simulink model "KERS_System_versione2"  (R2020a)
settings: Solver=VariableStepAuto  StartTime=0.0  StopTime=20  RelTol=1e-3
values from neighbouring files (symbols this model uses):
  Beta1 = 0.02    [Parameters.m]
  Beta2 = 0    [Parameters.m]
  Cx = 0.9    [Parameters.m]
  h = 0.1    [Parameters.m]
  Je = 0.3    [Kers_Energy_Characteristics.m]    (also in Kers_Energy_Characteristics_BiVariate.m; Parameters.m)
  Jf = 0.026    [Kers_Energy_Characteristics.m]    (also in Kers_Energy_Characteristics_BiVariate.m; Parameters.m)
  Jw = 1/2*(Rw^2*Mw)    (= 0.49005)    [Kers_Energy_Characteristics.m]    (also in Kers_Energy_Characteristics_BiVariate.m; Parameters.m)
  k = 0.01    [Parameters.m]
  M = 700    [Kers_Energy_Characteristics.m]    (also in Kers_Energy_Characteristics_BiVariate.m; Parameters.m)
  r_i = 0.05    [Parameters.m]
  r_o = 0.1    [Parameters.m]
  rho = Jeq^2*Jc/((Jc+Jeq)^2*gamma(i))    [Kers_Energy_Characteristics.m]    (also in Parameters.m = 1.2)
  rho_fw = 2267    [Parameters.m]
  Rw = 0.33    [Kers_Energy_Characteristics.m]    (also in Kers_Energy_Characteristics_BiVariate.m; Parameters.m)
  Sf = 1.5    [Parameters.m]
  tau1 = 1/3.08    (= 0.324675324675)    [Kers_Energy_Characteristics.m]    (also in Kers_Energy_Characteristics_BiVariate.m; Parameters.m)
  tau2 = 1/2.18    (= 0.45871559633)    [Kers_Energy_Characteristics.m]    (also in Kers_Energy_Characteristics_BiVariate.m; Parameters.m)
  tau3 = 1/1.63    (= 0.613496932515)    [Kers_Energy_Characteristics.m]    (also in Kers_Energy_Characteristics_BiVariate.m; Parameters.m)
  tau4 = 1/1.29    (= 0.77519379845)    [Kers_Energy_Characteristics.m]    (also in Kers_Energy_Characteristics_BiVariate.m; Parameters.m)
  tau5 = 1/1.03    (= 0.970873786408)    [Kers_Energy_Characteristics.m]    (also in Kers_Energy_Characteristics_BiVariate.m; Parameters.m)
  tau6 = 1/0.84    (= 1.19047619048)    [Kers_Energy_Characteristics.m]    (also in Kers_Energy_Characteristics_BiVariate.m; Parameters.m)
  tau7 = 1/0.69    (= 1.44927536232)    [Kers_Energy_Characteristics.m]    (also in Kers_Energy_Characteristics_BiVariate.m; Parameters.m)
  tauf = 1/4.38    (= 0.228310502283)    [Kers_Energy_Characteristics.m]    (also in Kers_Energy_Characteristics_BiVariate.m; Parameters.m)
  V1max = tauf*tau1*Rw*Wmax    (= 23.0528375734)    [Kers_Energy_Characteristics.m]    (also in Kers_Energy_Characteristics_BiVariate.m; Parameters.m)
  V2max = tauf*tau2*Rw*Wmax    (= 32.5700640945)    [Kers_Energy_Characteristics.m]    (also in Kers_Energy_Characteristics_BiVariate.m; Parameters.m)
  V3max = tauf*tau3*Rw*Wmax    (= 43.5599630221)    [Kers_Energy_Characteristics.m]    (also in Kers_Energy_Characteristics_BiVariate.m; Parameters.m)
  V4max = tauf*tau4*Rw*Wmax    (= 55.0408835085)    [Kers_Energy_Characteristics.m]    (also in Kers_Energy_Characteristics_BiVariate.m; Parameters.m)
  V5max = tauf*tau5*Rw*Wmax    (= 68.9346987631)    [Kers_Energy_Characteristics.m]    (also in Kers_Energy_Characteristics_BiVariate.m; Parameters.m)
  V6max = tauf*tau6*Rw*Wmax    (= 84.5270711024)    [Kers_Energy_Characteristics.m]    (also in Kers_Energy_Characteristics_BiVariate.m; Parameters.m)
  w_fw_max = 6283    [Parameters.m]
libraries: simulink x1
settings Model: Creator=Federico Kieffer  LastModifiedBy=Luca
settings SFSimCC: CustomCodeUndefinedFunction=UseInterfaceOnly

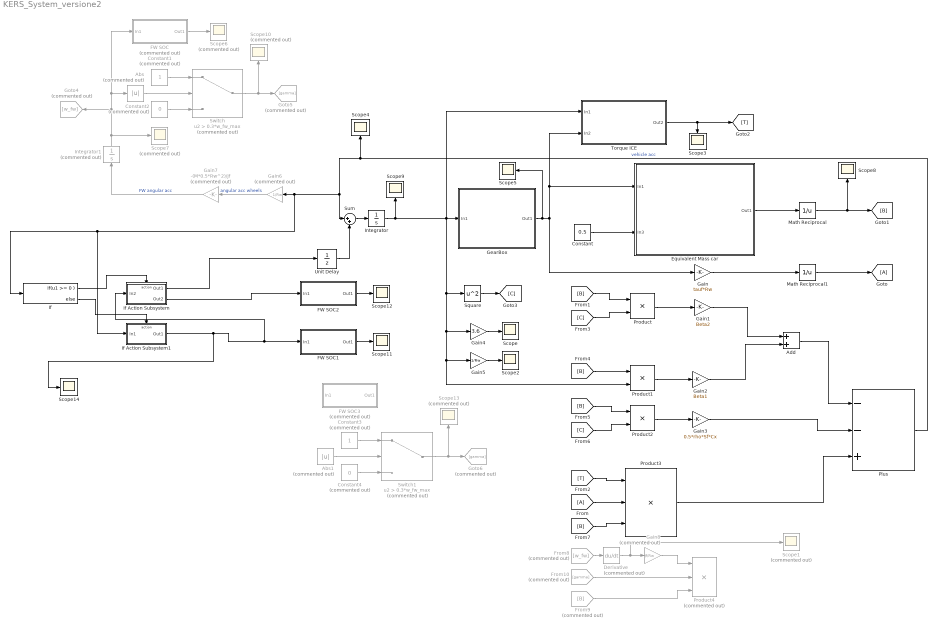
== system KERS_System_versione2 ==
  Abs : Abs  Commented=on
  Abs1 : Abs  Commented=on
  Add : Sum
  Constant : Constant  Value=0.5
  Constant1 : Constant  Commented=on
  Constant2 : Constant  Commented=on  Value=0
  Constant3 : Constant  Commented=on
  Constant4 : Constant  Commented=on  Value=0
  Derivative : Derivative  Commented=on
  Equivalent Mass car : Subsystem
      mask Display: image("f1.jpg")
  FW SOC : Subsystem  Commented=on
  FW SOC1 : Subsystem
  FW SOC2 : Subsystem
  FW SOC3 : Subsystem  Commented=on
  From10 : From  Commented=on  GotoTag=gamma
  From8 : From  Commented=on  GotoTag=w_fw
  From9 : From  Commented=on  GotoTag=B
  Gain : Gain  Gain=tauf*Rw
  Gain1 : Gain  Gain=Beta2
  Gain2 : Gain  Gain=Beta1
  Gain3 : Gain  Gain=0.5*rho*Sf*Cx
  Gain4 : Gain  Gain=3.6
  Gain5 : Gain  Gain=1/Rw
  Gain6 : Gain  Commented=on  Gain=1/Rw
  Gain7 : Gain  Commented=on  Gain=-(M*0.5*Rw^2)/Jf
  Gain8 : Gain  Commented=on  Gain=Jf/Rw
  GearBox : Subsystem
      mask Display: image("GearBox.jpg")
  Goto4 : Goto  Commented=on  GotoTag=w_fw
  Goto5 : Goto  Commented=on  GotoTag=gamma
  Goto6 : Goto  Commented=on  GotoTag=gamma
  If : If  IfExpression=u1 >= 0
  If Action Subsystem : Subsystem  TreatAsAtomicUnit=on
  If Action Subsystem1 : Subsystem  TreatAsAtomicUnit=on
  Integrator : Integrator  InitialCondition=42
  Integrator1 : Integrator  Commented=on
  Math Reciprocal : Math  Operator=reciprocal  SignedPower=on  SaturateOnIntegerOverflow=on
  Math Reciprocal1 : Math  Operator=reciprocal  SignedPower=on  SaturateOnIntegerOverflow=on
  Plus : Sum  Inputs=--+
  Product : Product
  Product1 : Product
  Product2 : Product
  Product3 : Product  Inputs=3
  Product4 : Product  Commented=on  Inputs=3
  Scope{,2..5,8..9,11..12,14} (10 alike) : Scope
  Scope{1,6..7,10,13} (5 alike) : Scope  Commented=on
  Square : Math  Operator=square  SignedPower=on  SaturateOnIntegerOverflow=on
  Sum : Sum  Inputs=|++
  Switch : Switch  Commented=on  Criteria=u2 > Threshold  Threshold=0.3*w_fw_max
  Switch1 : Switch  Commented=on  Criteria=u2 > Threshold  Threshold=0.3*w_fw_max
  Torque ICE : Subsystem
      mask Display: image("ICE.jpg")
  Unit Delay : UnitDelay  SampleTime=-1  HasFrameUpgradeWarning=on
  wires:
  Integrator/1 -> Gain4/1, Product1/2, Gain5/1, Square/1, GearBox/1(In1), Torque ICE/1(In1), Scope9/1
  GearBox/1(Out1) -> Gain/1, Torque ICE/2(In2), Equivalent Mass car/1(In1), Scope5/1
  Math Reciprocal/1 -> Scope8/1, [B]
  Gain/1 -> Math Reciprocal1/1
  Math Reciprocal1/1 -> [A]
  Square/1 -> [C]
  [B] -> Product/1
  [C] -> Product/2
  Product/1 -> Gain1/1
  [B] -> Product1/1
  Product1/1 -> Gain2/1
  Gain1/1 -> Add/1
  Gain2/1 -> Add/2
  [B] -> Product2/1
  [C] -> Product2/2
  Product2/1 -> Gain3/1
  [T] -> Product3/1
  [A] -> Product3/2
  [B] -> Product3/3
  Add/1 -> Plus/1
  Gain3/1 -> Plus/2
  Product3/1 -> Plus/3
  Plus/1 -> Scope4/1, Sum/1, If Action Subsystem1/1(In1), If/1, Gain6/1  "vehicle acc"
  Equivalent Mass car/1(Out1) -> Math Reciprocal/1
  Gain4/1 -> Scope/1
  Constant/1 -> Equivalent Mass car/2(In3)
  Gain5/1 -> Scope2/1
  Gain6/1 -> Gain7/1  "angular acc wheels"
  Gain7/1 -> Integrator1/1  "FW angular acc"
  Integrator1/1 -> Abs/1, FW SOC/1(In1), Goto4/1, Scope7/1
  Constant1/1 -> Switch/1
  Constant2/1 -> Switch/3
  Switch/1 -> Goto5/1, Scope10/1
  FW SOC/1(Out1) -> Scope6/1
  Torque ICE/1(Out2) -> Scope3/1, [T]
  Gain8/1 -> Product4/1
  From10/1 -> Product4/2
  From8/1 -> Derivative/1
  Derivative/1 -> Scope1/1, Gain8/1
  Abs/1 -> Switch/2
  From9/1 -> Product4/3
  FW SOC1/1(Out1) -> Scope11/1
  If Action Subsystem1/1(Out1) -> Scope14/1, If Action Subsystem/1(In2), FW SOC1/1(In1)
  FW SOC2/1(Out1) -> Scope12/1
  If Action Subsystem/2(Out2) -> FW SOC2/1(In1)
  If Action Subsystem/1(Out1) -> Unit Delay/1
  Sum/1 -> Integrator/1
  Unit Delay/1 -> Sum/2
  Constant4/1 -> Switch1/3
  Switch1/1 -> Goto6/1, Scope13/1
  Constant3/1 -> Switch1/1
  Abs1/1 -> Switch1/2
  If/1 -> If Action Subsystem/Action
  If/2 -> If Action Subsystem1/Action

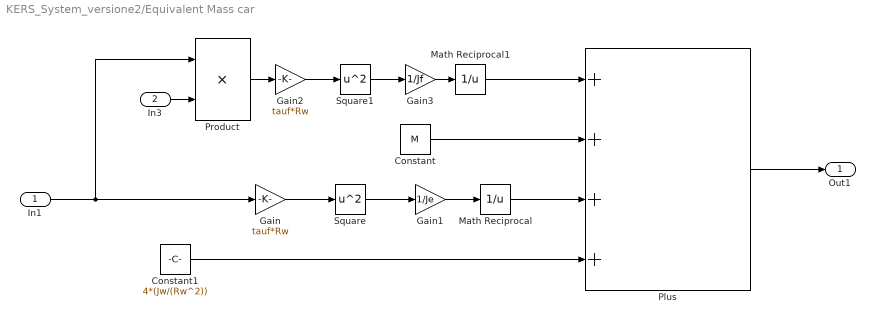
== system KERS_System_versione2/Equivalent Mass car ==
  In1 : Inport
  In3 : Inport  Port=2
  Constant : Constant  Value=M
  Constant1 : Constant  Value=4*(Jw/(Rw^2))
  Gain : Gain  Gain=tauf*Rw
  Gain1 : Gain  Gain=1/Je
  Gain2 : Gain  Gain=tauf*Rw
  Gain3 : Gain  Gain=1/Jf
  Math Reciprocal : Math  Operator=reciprocal  SignedPower=on  SaturateOnIntegerOverflow=on
  Math Reciprocal1 : Math  Operator=reciprocal  SignedPower=on  SaturateOnIntegerOverflow=on
  Plus : Sum  Inputs=++++
  Product : Product
  Square : Math  Operator=square  SignedPower=on  SaturateOnIntegerOverflow=on
  Square1 : Math  Operator=square  SignedPower=on  SaturateOnIntegerOverflow=on
  Out1 : Outport  VectorParamsAs1DForOutWhenUnconnected=off
  wires:
  In1/1 -> Gain/1, Product/1
  Gain/1 -> Square/1
  Square/1 -> Gain1/1
  Gain1/1 -> Math Reciprocal/1
  Math Reciprocal/1 -> Plus/3
  Constant/1 -> Plus/2
  Plus/1 -> Out1/1
  Constant1/1 -> Plus/4
  Product/1 -> Gain2/1
  Gain2/1 -> Square1/1
  Square1/1 -> Gain3/1
  Gain3/1 -> Math Reciprocal1/1
  In3/1 -> Product/2
  Math Reciprocal1/1 -> Plus/1

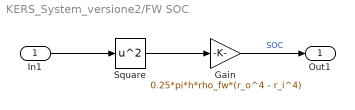
== system KERS_System_versione2/FW SOC ==
  In1 : Inport
  Gain : Gain  Gain=0.25*pi*h*rho_fw*(r_o^4 - r_i^4)
  Square : Math  Operator=square  SaturateOnIntegerOverflow=on
  Out1 : Outport
  wires:
  In1/1 -> Square/1
  Square/1 -> Gain/1
  Gain/1 -> Out1/1  "SOC"

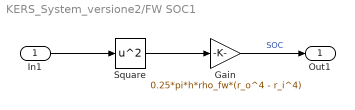
== system KERS_System_versione2/FW SOC1 ==
  In1 : Inport
  Gain : Gain  Gain=0.25*pi*h*rho_fw*(r_o^4 - r_i^4)
  Square : Math  Operator=square  SaturateOnIntegerOverflow=on
  Out1 : Outport
  wires:
  In1/1 -> Square/1
  Square/1 -> Gain/1
  Gain/1 -> Out1/1  "SOC"

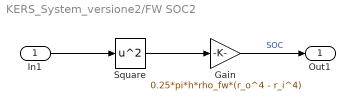
== system KERS_System_versione2/FW SOC2 ==
  In1 : Inport
  Gain : Gain  Gain=0.25*pi*h*rho_fw*(r_o^4 - r_i^4)
  Square : Math  Operator=square  SaturateOnIntegerOverflow=on
  Out1 : Outport
  wires:
  In1/1 -> Square/1
  Square/1 -> Gain/1
  Gain/1 -> Out1/1  "SOC"

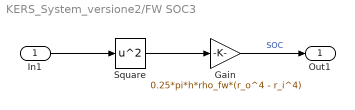
== system KERS_System_versione2/FW SOC3 ==
  In1 : Inport
  Gain : Gain  Gain=0.25*pi*h*rho_fw*(r_o^4 - r_i^4)
  Square : Math  Operator=square  SaturateOnIntegerOverflow=on
  Out1 : Outport
  wires:
  In1/1 -> Square/1
  Square/1 -> Gain/1
  Gain/1 -> Out1/1  "SOC"

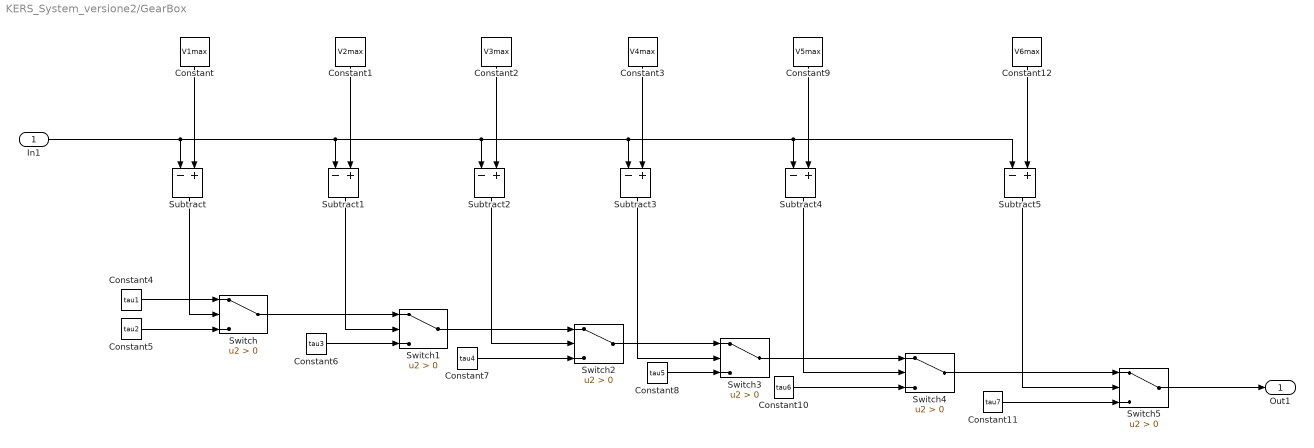
== system KERS_System_versione2/GearBox ==
  In1 : Inport
  Constant : Constant  Value=V1max
  Constant1 : Constant  Value=V2max
  Constant10 : Constant  Value=tau6
  Constant11 : Constant  Value=tau7
  Constant12 : Constant  Value=V6max
  Constant2 : Constant  Value=V3max
  Constant3 : Constant  Value=V4max
  Constant4 : Constant  Value=tau1
  Constant5 : Constant  Value=tau2
  Constant6 : Constant  Value=tau3
  Constant7 : Constant  Value=tau4
  Constant8 : Constant  Value=tau5
  Constant9 : Constant  Value=V5max
  Subtract{,1..5} (6 alike) : Sum  Inputs=-+
  Switch{,1..5} (6 alike) : Switch  Criteria=u2 > Threshold
  Out1 : Outport  VectorParamsAs1DForOutWhenUnconnected=off
  wires:
  Constant/1 -> Subtract/2
  In1/1 -> Subtract/1, Subtract1/1, Subtract2/1, Subtract3/1, Subtract4/1, Subtract5/1
  Constant1/1 -> Subtract1/2
  Constant2/1 -> Subtract2/2
  Constant3/1 -> Subtract3/2
  Subtract/1 -> Switch/2
  Constant4/1 -> Switch/1
  Constant5/1 -> Switch/3
  Subtract1/1 -> Switch1/2
  Switch/1 -> Switch1/1
  Constant6/1 -> Switch1/3
  Switch1/1 -> Switch2/1
  Subtract2/1 -> Switch2/2
  Constant7/1 -> Switch2/3
  Switch2/1 -> Switch3/1
  Subtract3/1 -> Switch3/2
  Constant8/1 -> Switch3/3
  Constant9/1 -> Subtract4/2
  Subtract4/1 -> Switch4/2
  Switch3/1 -> Switch4/1
  Constant10/1 -> Switch4/3
  Constant11/1 -> Switch5/3
  Constant12/1 -> Subtract5/2
  Subtract5/1 -> Switch5/2
  Switch4/1 -> Switch5/1
  Switch5/1 -> Out1/1

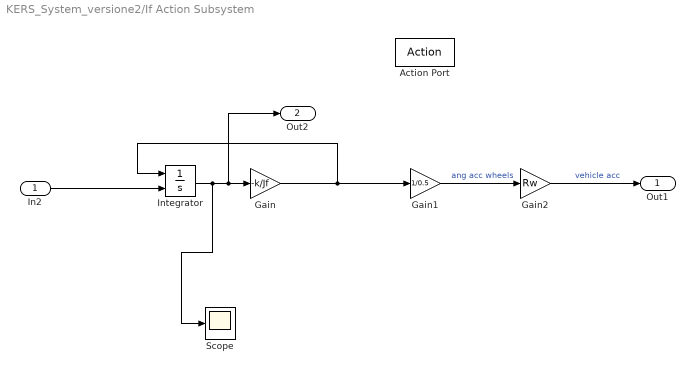
== system KERS_System_versione2/If Action Subsystem ==
  In2 : Inport
  Action Port : ActionPort  ActionPortLabel=if(u1 >= 0 )
  Gain : Gain  Gain=-k/Jf
  Gain1 : Gain  Gain=1/0.5
  Gain2 : Gain  Gain=Rw
  Integrator : Integrator  InitialConditionSource=external  InitialCondition=w_fw_max
  Scope : Scope
  Out1 : Outport
  Out2 : Outport  Port=2
  wires:
  Gain1/1 -> Gain2/1  "ang acc wheels"
  Gain2/1 -> Out1/1  "vehicle acc"
  Integrator/1 -> Scope/1, Out2/1, Gain/1
  Gain/1 -> Gain1/1, Integrator/1
  In2/1 -> Integrator/2

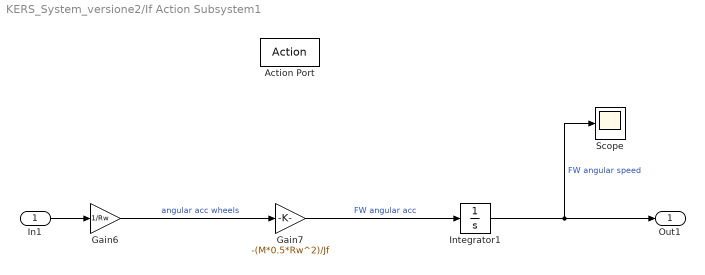
== system KERS_System_versione2/If Action Subsystem1 ==
  In1 : Inport
  Action Port : ActionPort  ActionPortLabel=else
  Gain6 : Gain  Gain=1/Rw
  Gain7 : Gain  Gain=-(M*0.5*Rw^2)/Jf
  Integrator1 : Integrator
  Scope : Scope
  Out1 : Outport
  wires:
  Gain7/1 -> Integrator1/1  "FW angular acc"
  Gain6/1 -> Gain7/1  "angular acc wheels"
  Integrator1/1 -> Scope/1, Out1/1  "FW angular speed"
  In1/1 -> Gain6/1

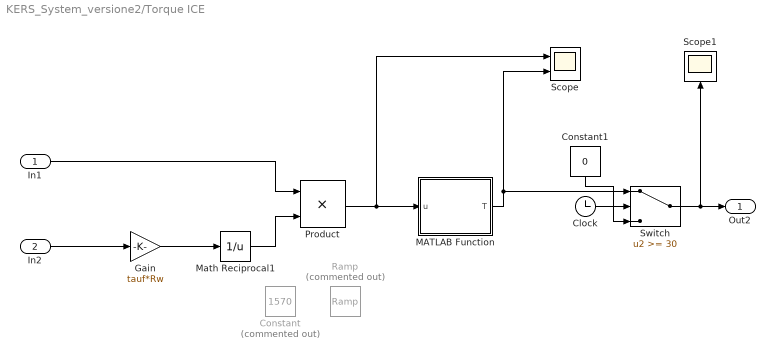
== system KERS_System_versione2/Torque ICE ==
  In1 : Inport
  In2 : Inport  Port=2
  Clock : Clock
  Constant : Constant  Commented=on  Value=1570
  Constant1 : Constant  Value=0
  Gain : Gain  Gain=tauf*Rw
  MATLAB Function : MATLAB Function  TreatAsAtomicUnit=on
  Math Reciprocal1 : Math  Operator=reciprocal  SignedPower=on  SaturateOnIntegerOverflow=on
  Product : Product
  Ramp : simulink/Sources/Ramp  Commented=on  slope=1  start=0  InitialOutput=0
  Scope : Scope  NumInputPorts=2
  Scope1 : Scope
  Switch : Switch  Threshold=30
  Out2 : Outport  VectorParamsAs1DForOutWhenUnconnected=off
  wires:
  In2/1 -> Gain/1
  Gain/1 -> Math Reciprocal1/1
  Math Reciprocal1/1 -> Product/2
  In1/1 -> Product/1
  Product/1 -> MATLAB Function/1(u), Scope/1
  MATLAB Function/1(T) -> Switch/1, Scope/2
  Switch/1 -> Out2/1, Scope1/1
  Clock/1 -> Switch/2
  Constant1/1 -> Switch/3

== matlab function KERS_System_versione2/Torque ICE/MATLAB Function ==
  data: u input; T output
function T = TorqueICE(u)

%T = a0+a1*u+a2*(u^2)+a3*(u^3);
T = 88.48+1.41*u-(8.36e-4)*(u^2);
